simulink model "lab3gravityBA"  (R2023b)
settings: Solver=VariableStepAuto  StartTime=0.0  StopTime=10.0  RelTol=1e-3
values from neighbouring files (symbols this model uses):
  par = [3, 2, 1, 0.6, 5.0, 5.0, 9.81]    [lab3init.m]
settings Model: Creator=rpl  LastModifiedBy=rpl

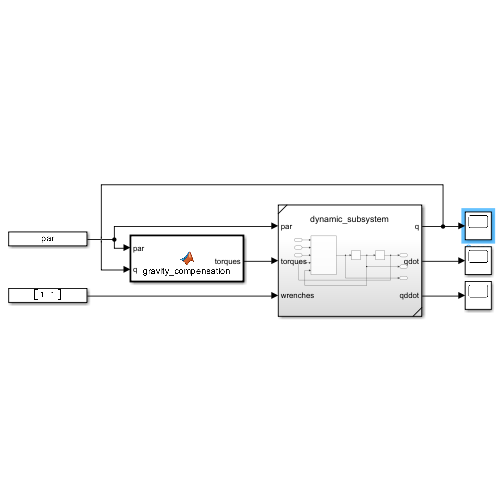
[thumbnail: Simulink's stored preview of the top-level diagram]
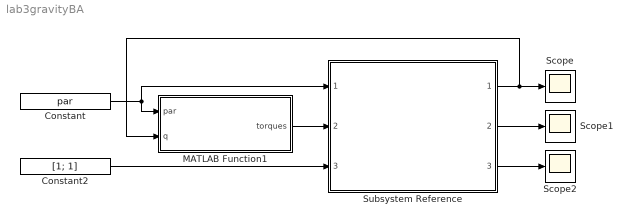
== system lab3gravityBA ==
  Constant : Constant  Value=par
  Constant2 : Constant  Value=[1; 1]
  MATLAB Function1 : MATLAB Function  TreatAsAtomicUnit=on
  Scope : Scope
  Scope1 : Scope
  Scope2 : Scope
  Subsystem Reference : Subsystem  ReferencedSubsystem=dynamic_subsystem
  wires:
  Constant/1 -> MATLAB Function1/1(par), Subsystem Reference/1
  Constant2/1 -> Subsystem Reference/3
  MATLAB Function1/1(torques) -> Subsystem Reference/2
  Subsystem Reference/1 -> Scope/1, MATLAB Function1/2(q)
  Subsystem Reference/2 -> Scope1/1
  Subsystem Reference/3 -> Scope2/1

== matlab function lab3gravityBA/MATLAB Function1 ==
  data: par input; q input; torques output
function torques = gravity_compensation(par, q)

    m1 = par(1);
    m2 = par(2);
    l1 = par(3);
    l2 = par(4);
    g = par(7);

    % sines and cosines
    cq1 = cos(q(1));
    cq12 = cos(q(1)+q(2));
    
    % Calculate g(q)
    g = [(m1+m2)*l1*g*cq1+m2*g*l2*cq12;
          m2*g*l2*cq12];

    torques = g;
